simulink model "FOC_control"  (R2019a)
settings: Solver=VariableStepAuto  StartTime=0.0  StopTime=10.0  RelTol=1e-3
undefined symbols (not defined in the file or in its folder): PWM_EN, sf, Ts
libraries: nesl_utility x13, ee_lib x10, fl_lib x10, msbAdcArchitectures x6, eeTransforms x4, eePmsmCurrentController x1, eePmsmCurrentReferenceGen x1, eePwmGeneratorTwoLevel x1, eeVelocityController x1, simulink x1
(part 2 of 3)

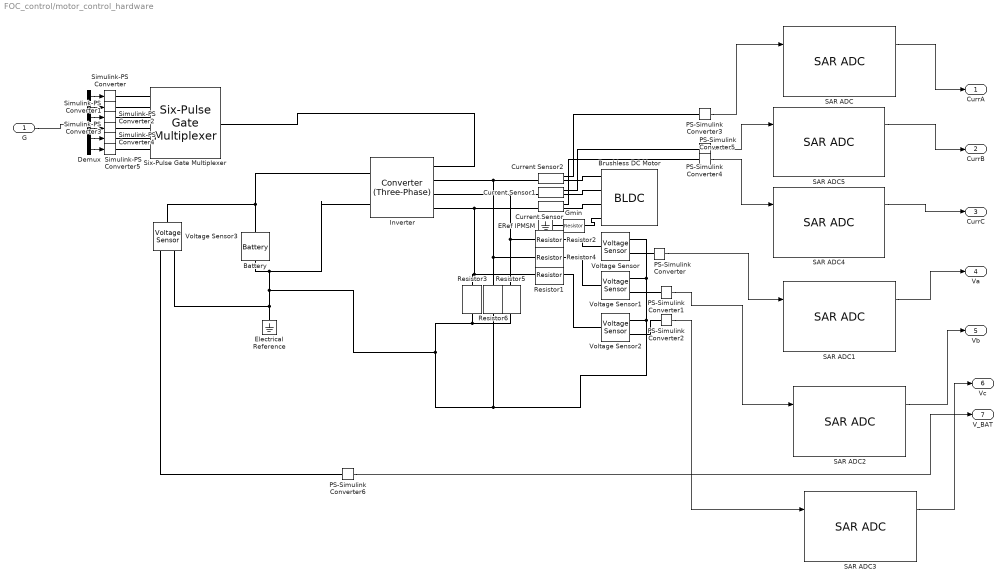
== system FOC_control/motor_control_hardware  ==
  G : Inport  Tag=G
  Battery : ee_lib/Sources/Battery  Vnom=43.2 V  R1=2 Ohm  prm_AH=1  AH=50 hr*A  V1=11.5 V  AH1=25 hr*A  prm_R2=1  R2=2000 Ohm  prm_dyn=1  Rp1=0.005 Ohm  tau1=30 s  Rp2=0.005 Ohm  tau2=30 s  Rp3=0.005 Ohm  tau3=30 s  Rp4=0.005 Ohm  tau4=30 s  Rp5=0.005 Ohm  tau5=30 s  prm_fade=1  N_fade=100  AH_fade=45 hr*A  R1_fade=2.02 Ohm  V1_fade=10.35 V  i_specify=off  i_priority=None  i=0 A  i_nominal_specify=off  i_nominal_unit=A  i_nominal_value=1  v_specify=off  v_priority=None  v=0 V  v_nominal_specify=off  v_nominal_unit=V  v_nominal_value=1  charge_specify=off  charge_priority=High  charge=50 hr*A  charge_nominal_specify=off  charge_nominal_unit=hr*A  charge_nominal_value=1  num_cycles_specify=off  num_cycles_priority=High  num_cycles=0  num_cycles_nominal_specify=off  num_cycles_nominal_unit=1  num_cycles_nominal_value=1  thermal_mass=30000 J/K  Tmeas=298.15 K  Vnom_T2=12 V  R1_T2=2.2 Ohm  V1_T2=11.4 V  R2_T2=2200 Ohm  Rp1_T2=0.005 Ohm  tau1_T2=30 s  Rp2_T2=0.005 Ohm  tau2_T2=30 s  Rp3_T2=0.005 Ohm  tau3_T2=30 s  Rp4_T2=0.005 Ohm  tau4_T2=30 s  Rp5_T2=0.005 Ohm  tau5_T2=30 s  Tmeas2=273.15 K  temperature_specify=off  temperature_priority=High  temperature=298.15 K  temperature_nominal_specify=off  temperature_nominal_unit=K  temperature_nominal_value=1
      settings: SourceProductName=Simscape Electrical
  Brushless DC Motor : ee_lib/Electromechanical/Permanent Magnet/BLDC  rotor_param=1  pm_flux_linkage=0.03 Wb  theta_constant=pi / 12 rad  emf_max=9.6 V  DphiDtheta_tab=[0, -.1528, -.1528, .1528, .1528, 0] Wb/rad  back_emf_tab=[0, -9.6, -9.6, 9.6, 9.6, 0] V  rotor_angle_tab=[0, 7.5, 22.5, 37.5, 52.5, 60] deg  w_meas=600 rpm  nPolePairs=6  stator_param=1  Ld=0.00022 H  Lq=0.00022 H  L0=0.00016 H  Ls=0.0002 H  Lm=0 H  Ms=0.00002 H  Rs=0.013 Ohm  zero_sequence=ee.enum.park.zerosequence.include  J=0.01 kg*m^2  lam=0 N*m/(rad/s)  axes_param=2  i_d_specify=off  i_d_priority=None  i_d=0 A  i_d_nominal_specify=off  i_d_nominal_unit=A  i_d_nominal_value=1  i_q_specify=off  i_q_priority=None  i_q=0 A  i_q_nominal_specify=off  i_q_nominal_unit=A  i_q_nominal_value=1  torque_specify=off  torque_priority=None  torque=0 N*m  torque_nominal_specify=off  torque_nominal_unit=N*m  torque_nominal_value=1  angular_velocity_specify=off  angular_velocity_priority=High  angular_velocity=0 rpm  angular_velocity_nominal_specify=off  angular_velocity_nominal_unit=rpm  angular_velocity_nominal_value=1  angular_position_specify=off  angular_position_priority=High  angular_position=0 deg  angular_position_nominal_specify=off  angular_position_nominal_unit=deg  angular_position_nominal_value=1
      settings: SourceProductName=Simscape Electrical  SourceProductBaseCode=PS
  Current Sensor : fl_lib/Electrical/Electrical Sensors/Current Sensor
  Current Sensor1 : fl_lib/Electrical/Electrical Sensors/Current Sensor
  Current Sensor2 : fl_lib/Electrical/Electrical Sensors/Current Sensor
  Demux : Demux  Outputs=6
  ERef IPMSM : fl_lib/Electrical/Electrical Elements/Electrical Reference
      settings: SourceProductName=Foundation Library
  Electrical Reference : fl_lib/Electrical/Electrical Elements/Electrical Reference
  Gmin : fl_lib/Electrical/Electrical Elements/Resistor  R=1e9 Ohm  i_specify=off  i_priority=High  i=0 A  i_nominal_specify=off  i_nominal_unit=A  i_nominal_value=1  v_specify=off  v_priority=High  v=0 V  v_nominal_specify=off  v_nominal_unit=V  v_nominal_value=1
      settings: SourceProductName=Foundation Library
  Inverter : ee_lib/Semiconductors & Converters/Converters/Converter (Three-Phase)  device_type=4  Vf=0.8 V  Ron=0.001 Ohm  Rds=0.001 Ohm  Goff=1e-5 1/Ohm  Vth=0.5 V  Vgt=1 V  Vgt_off=-1 V  Ih=1 A  diode_param=2  diode_Vf=0.8 V  diode_Ron=0.001 Ohm  diode_Goff=1e-5 1/Ohm  diode_C=50 nF  diode_iRM=-235 A  diode_iF=300 A  diode_idot=-50 A/us  diode_trr_param=1  diode_trr_factor=3  diode_trr=15 us  diode_Qrr=1.5e+3 s*uA  snubber_type=0  Rs=0.1 Ohm  Cs=1e-7 F
      settings: SourceProductName=Simscape Electrical  SourceProductBaseCode=PS
  PS-Simulink Converter{,1..6} (7 alike) : nesl_utility/PS-Simulink Converter  PhysicalDomain=network_engine_domain  SubClassName=ps_output  LeftPortType=input  RightPortType=output  PseudoPeriodic=off  Frequencies=[]  Unit=1  AffineConversion=off
  Resistor1 : ee_lib/Passive/Resistor  R=39000 Ohm  R_tol=1  enable_R_tol=1  tol_distribution=1  nSigma=4  enable_operating_limits=0  operating_limit_action=2  max_working_voltage=100 V  power_rating=1 W  enable_faults=0  fault_action=1  R_faulted=inf Ohm  enable_temporal_fault=0  t_fault=1 s  enable_behavioral_fault=0  max_permissible_current=1 A  t_fail_on_current=1 s  noise_mode=0  sample_time=1e-3 s  repeatability=1  auto_seed=797911566  user_seed=0  Tdevice=25 degC  alpha=3.93e-3 1/K  Tmeas=25 degC  thermal_mass=100 J/K  power_derating_T1=70 degC  power_derating_T2=155 degC  operating_temperature_range_vec=[-50, 150] degC  temperature_specify=off  temperature_priority=High  temperature=298.15 K  temperature_nominal_specify=off  temperature_nominal_unit=K  temperature_nominal_value=1
      settings: SourceProductName=Simscape Electrical
  Resistor2 : ee_lib/Passive/Resistor  R=39000 Ohm  R_tol=1  enable_R_tol=1  tol_distribution=1  nSigma=4  enable_operating_limits=0  operating_limit_action=2  max_working_voltage=100 V  power_rating=1 W  enable_faults=0  fault_action=1  R_faulted=inf Ohm  enable_temporal_fault=0  t_fault=1 s  enable_behavioral_fault=0  max_permissible_current=1 A  t_fail_on_current=1 s  noise_mode=0  sample_time=1e-3 s  repeatability=1  auto_seed=770095556  user_seed=0  Tdevice=25 degC  alpha=3.93e-3 1/K  Tmeas=25 degC  thermal_mass=100 J/K  power_derating_T1=70 degC  power_derating_T2=155 degC  operating_temperature_range_vec=[-50, 150] degC  temperature_specify=off  temperature_priority=High  temperature=298.15 K  temperature_nominal_specify=off  temperature_nominal_unit=K  temperature_nominal_value=1
      settings: SourceProductName=Simscape Electrical
  Resistor3 : ee_lib/Passive/Resistor  R=2200 Ohm  R_tol=1  enable_R_tol=1  tol_distribution=1  nSigma=4  enable_operating_limits=0  operating_limit_action=2  max_working_voltage=100 V  power_rating=1 W  enable_faults=0  fault_action=1  R_faulted=inf Ohm  enable_temporal_fault=0  t_fault=1 s  enable_behavioral_fault=0  max_permissible_current=1 A  t_fail_on_current=1 s  noise_mode=0  sample_time=1e-3 s  repeatability=1  auto_seed=829099697  user_seed=0  Tdevice=25 degC  alpha=3.93e-3 1/K  Tmeas=25 degC  thermal_mass=100 J/K  power_derating_T1=70 degC  power_derating_T2=155 degC  operating_temperature_range_vec=[-50, 150] degC  temperature_specify=off  temperature_priority=High  temperature=298.15 K  temperature_nominal_specify=off  temperature_nominal_unit=K  temperature_nominal_value=1
      settings: SourceProductName=Simscape Electrical
  Resistor4 : ee_lib/Passive/Resistor  R=39000 Ohm  R_tol=1  enable_R_tol=1  tol_distribution=1  nSigma=4  enable_operating_limits=0  operating_limit_action=2  max_working_voltage=100 V  power_rating=1 W  enable_faults=0  fault_action=1  R_faulted=inf Ohm  enable_temporal_fault=0  t_fault=1 s  enable_behavioral_fault=0  max_permissible_current=1 A  t_fail_on_current=1 s  noise_mode=0  sample_time=1e-3 s  repeatability=1  auto_seed=1467350256  user_seed=0  Tdevice=25 degC  alpha=3.93e-3 1/K  Tmeas=25 degC  thermal_mass=100 J/K  power_derating_T1=70 degC  power_derating_T2=155 degC  operating_temperature_range_vec=[-50, 150] degC  temperature_specify=off  temperature_priority=High  temperature=298.15 K  temperature_nominal_specify=off  temperature_nominal_unit=K  temperature_nominal_value=1
      settings: SourceProductName=Simscape Electrical
  Resistor5 : ee_lib/Passive/Resistor  R=2200 Ohm  R_tol=1  enable_R_tol=1  tol_distribution=1  nSigma=4  enable_operating_limits=0  operating_limit_action=2  max_working_voltage=100 V  power_rating=1 W  enable_faults=0  fault_action=1  R_faulted=inf Ohm  enable_temporal_fault=0  t_fault=1 s  enable_behavioral_fault=0  max_permissible_current=1 A  t_fail_on_current=1 s  noise_mode=0  sample_time=1e-3 s  repeatability=1  auto_seed=1289282186  user_seed=0  Tdevice=25 degC  alpha=3.93e-3 1/K  Tmeas=25 degC  thermal_mass=100 J/K  power_derating_T1=70 degC  power_derating_T2=155 degC  operating_temperature_range_vec=[-50, 150] degC  temperature_specify=off  temperature_priority=High  temperature=298.15 K  temperature_nominal_specify=off  temperature_nominal_unit=K  temperature_nominal_value=1
      settings: SourceProductName=Simscape Electrical
  Resistor6 : ee_lib/Passive/Resistor  R=2200 Ohm  R_tol=1  enable_R_tol=1  tol_distribution=1  nSigma=4  enable_operating_limits=0  operating_limit_action=2  max_working_voltage=100 V  power_rating=1 W  enable_faults=0  fault_action=1  R_faulted=inf Ohm  enable_temporal_fault=0  t_fault=1 s  enable_behavioral_fault=0  max_permissible_current=1 A  t_fail_on_current=1 s  noise_mode=0  sample_time=1e-3 s  repeatability=1  auto_seed=4006765953  user_seed=0  Tdevice=25 degC  alpha=3.93e-3 1/K  Tmeas=25 degC  thermal_mass=100 J/K  power_derating_T1=70 degC  power_derating_T2=155 degC  operating_temperature_range_vec=[-50, 150] degC  temperature_specify=off  temperature_priority=High  temperature=298.15 K  temperature_nominal_specify=off  temperature_nominal_unit=K  temperature_nominal_value=1
      settings: SourceProductName=Simscape Electrical
  SAR ADC : msbAdcArchitectures/SAR ADC  DACVoltages=[-5:5]  DACINLVoltages=tanh([-5:5])  NBits=12  InputRange=[-3.3 3.3]  ExtStartClk=on  StartFreq=10e3  StartClkJitter=0  SARFreq=2e7  OutDataType=BinaryVector  EnableImp=on  OffsetError=1  GainError=2  GainErrorUnit=LSB  INL=[1 1.00048851978505 1.0009770395701 1.00146555935515 1.00195407914021 1.00244259892526 1.00293111871031 1.00341963849536 1.00390815828041 1.00439667806546 1.00488519785051 1.00537371763556 1.00586223742062 1.00635075720567 1.00683927699072 1.00732779677577 1.00781631656082 1.00830483634587 1.00879335613092 1.00928187591597 1.00977039570103 1.01025891548608 1.01074743527113 1.01123595505618 1.01172447484123 1.01221299462628 1.01270151441133 1.01319003419638 1.01367855398144 1.01416707376649 1.01465559355154 1.01514411333659 1.01563263312164 1.01612115290669 1.01660967269174 1.01709819247679 1.01758671226185 1.0180752320469 1.01856375183195 1.019052271617 1.01954079140205 1.0200293111871 1.02051783097215 1.0210063507572 1.02149487054226 1.02198339032731 1.02247191011236 1.02296042989741 1.02344894968246 1.02393746946751 1.02442598925256 1.02491450903761 1.02540302882267 1.02589154860772 1.02638006839277 1.02686858817782 1.02735710796287 1.02784562774792 1.02833414753297 1.02882266731802 1.02931118710308 1.02979970688813 1.03028822667318 1.03077674645823 1.03126526624328 1.03175378602833 1.03224230581338 1.03273082559843 1.03321934538349 1.03370786516854 1.03419638495359 1.03468490473864 1.03517342452369 1.03566194430874 1.03615046409379 1.03663898387885 1.0371275036639 1.03761602344895 1.038104543234 1.03859306301905 1.0390815828041 1.03957010258915 1.0400586223742 1.04054714215926 1.04103566194431 1.04152418172936 1.04201270151441 1.04250122129946 1.04298974108451 1.04347826086956 1.04396678065461 1.04445530043967 1.04494382022472 1.04543234000977 1.04592085979482 1.04640937957987 1.04689789936492 1.04738641914997 1.04787493893502 1.04836345872008 1.04885197850513 1.04934049829018 1.04982901807523 1.05031753786028 1.05080605764533 1.05129457743038 1.05178309721543 1.05227161700049 1.05276013678554 1.05324865657059 1.05373717635564 1.05422569614069 1.05471421592574 1.05520273571079 1.05569125549584 1.0561797752809 1.05666829506595 1.057156814851 1.05764533463605 1.0581338544211 1.05862237420615 1.0591108939912 1.05959941377625 1.06008793356131 1.06057645334636 1.06106497313141 1.06155349291646 1.06204201270151 1.06253053248656 1.06301905227161 1.06350757205666 1.06399609184172 1.06448461162677 1.06497313141182 1.06546165119687 1.06595017098192 1.06643869076697 1.06692721055202 1.06741573033707 1.06790425012213 1.06839276990718 1.06888128969223 1.06936980947728 1.06985832926233 1.07034684904738 1.07083536883243 1.07132388861748 1.07181240840254 1.07230092818759 1.07278944797264 1.07327796775769 1.07376648754274 1.07425500732779 1.07474352711284 1.0752320468979 1.07572056668295 1.076209086468 1.07669760625305 1.0771861260381 1.07767464582315 1.0781631656082 1.07865168539325 1.07914020517831 1.07962872496336 1.08011724474841 1.08060576453346 1.08109428431851 1.08158280410356 1.08207132388861 1.08255984367366 1.08304836345872 1.08353688324377 1.08402540302882 1.08451392281387 1.08500244259892 1.08549096238397 1.08597948216902 1.08646800195407 1.08695652173913 1.08744504152418 1.08793356130923 1.08842208109428 1.08891060087933 1.08939912066438 1.08988764044943 1.09037616023448 1.09086468001954 1.09135319980459 1.09184171958964 1.09233023937469 1.09281875915974 1.09330727894479 1.09379579872984 1.09428431851489 1.09477283829995 1.095261358085 1.09574987787005 1.0962383976551 1.09672691744015 1.0972154372252 1.09770395701025 1.0981924767953 1.09868099658036 1.09916951636541 1.09965803615046 1.10014655593551 1.10063507572056 1.10112359550561 1.10161211529066 1.10210063507571 1.10258915486077 1.10307767464582 1.10356619443087 1.10405471421592 1.10454323400097 1.10503175378602 1.10552027357107 1.10600879335612 1.10649731314118 1.10698583292623 1.10747435271128 1.10796287249633 1.10845139228138 1.10893991206643 1.10942843185148 1.10991695163654 1.11040547142159 1.11089399120664 1.11138251099169 1.11187103077674 1.11235955056179 1.11284807034684 1.11333659013189 1.11382510991695 1.114313629702 1.11480214948705 1.1152906692721 ...(+65139 chars)]
      settings: SourceProductName=Mixed-Signal Blockset  SourceProductBaseCode=AM
  SAR ADC{1..5} (5 alike) : msbAdcArchitectures/SAR ADC  DACVoltages=[-5:5]  DACINLVoltages=tanh([-5:5])  NBits=8  InputRange=[-1 1]  ExtStartClk=on  StartFreq=10e3  StartClkJitter=0  SARFreq=2e7  OutDataType=BinaryVector  EnableImp=on  OffsetError=1  GainError=2  GainErrorUnit=LSB  INL=[1 1.00787401574803 1.01574803149606 1.02362204724409 1.03149606299213 1.03937007874016 1.04724409448819 1.05511811023622 1.06299212598425 1.07086614173228 1.07874015748031 1.08661417322835 1.09448818897638 1.10236220472441 1.11023622047244 1.11811023622047 1.1259842519685 1.13385826771654 1.14173228346457 1.1496062992126 1.15748031496063 1.16535433070866 1.17322834645669 1.18110236220473 1.18897637795276 1.19685039370079 1.20472440944882 1.21259842519685 1.22047244094488 1.22834645669291 1.23622047244094 1.24409448818898 1.25196850393701 1.25984251968504 1.26771653543307 1.2755905511811 1.28346456692913 1.29133858267716 1.2992125984252 1.30708661417323 1.31496062992126 1.32283464566929 1.33070866141733 1.33858267716536 1.34645669291339 1.35433070866141 1.36220472440945 1.37007874015748 1.37795275590551 1.38582677165354 1.39370078740158 1.40157480314961 1.40944881889764 1.41732283464567 1.4251968503937 1.43307086614173 1.44094488188976 1.44881889763779 1.45669291338583 1.46456692913386 1.47244094488189 1.48031496062992 1.48818897637796 1.49606299212599 1.50393700787401 1.51181102362204 1.51968503937007 1.5275590551181 1.53543307086615 1.54330708661418 1.55118110236221 1.55905511811024 1.56692913385827 1.5748031496063 1.58267716535433 1.59055118110236 1.5984251968504 1.60629921259843 1.61417322834646 1.62204724409449 1.62992125984252 1.63779527559055 1.64566929133858 1.65354330708661 1.66141732283465 1.66929133858268 1.67716535433071 1.68503937007874 1.69291338582677 1.7007874015748 1.70866141732283 1.71653543307086 1.7244094488189 1.73228346456693 1.74015748031496 1.74803149606299 1.75590551181102 1.76377952755905 1.77165354330708 1.77952755905511 1.78740157480316 1.79527559055119 1.80314960629921 1.81102362204724 1.81889763779527 1.8267716535433 1.83464566929133 1.84251968503936 1.85039370078741 1.85826771653544 1.86614173228347 1.8740157480315 1.88188976377953 1.88976377952756 1.89763779527559 1.90551181102362 1.91338582677166 1.92125984251969 1.92913385826772 1.93700787401575 1.94488188976378 1.95275590551181 1.96062992125984 1.96850393700787 1.97637795275591 1.98425196850394 1.99212598425197 2 2.00787401574803 2.01574803149606 2.02362204724409 2.03149606299212 2.03937007874015 2.04724409448818 2.05511811023621 2.06299212598427 2.0708661417323 2.07874015748033 2.08661417322836 2.09448818897638 2.10236220472441 2.11023622047244 2.11811023622047 2.1259842519685 2.13385826771653 2.14173228346456 2.14960629921259 2.15748031496062 2.16535433070865 2.17322834645668 2.18110236220471 2.18897637795277 2.1968503937008 2.20472440944883 2.21259842519686 2.22047244094489 2.22834645669292 2.23622047244095 2.24409448818898 2.25196850393701 2.25984251968504 2.26771653543307 2.2755905511811 2.28346456692913 2.29133858267716 2.29921259842519 2.30708661417322 2.31496062992127 2.3228346456693 2.33070866141733 2.33858267716536 2.34645669291339 2.35433070866142 2.36220472440945 2.37007874015748 2.37795275590551 2.38582677165354 2.39370078740157 2.4015748031496 2.40944881889763 2.41732283464566 2.42519685039369 2.43307086614172 2.44094488188978 2.44881889763781 2.45669291338584 2.46456692913387 2.4724409448819 2.48031496062993 2.48818897637796 2.49606299212599 2.50393700787401 2.51181102362204 2.51968503937007 2.5275590551181 2.53543307086613 2.54330708661416 2.55118110236219 2.55905511811022 2.56692913385828 2.57480314960631 2.58267716535434 2.59055118110237 2.5984251968504 2.60629921259843 2.61417322834646 2.62204724409449 2.62992125984252 2.63779527559055 2.64566929133858 2.65354330708661 2.66141732283464 2.66929133858267 2.6771653543307 2.68503937007873 2.69291338582678 2.70078740157481 2.70866141732284 2.71653543307087 2.7244094488189 2.73228346456693 2.74015748031496 2.74803149606299 2.75590551181102 2.76377952755905 2.77165354330708 2.77952755905511 2.78740157480314 2.79527559055117 2.8031496062992 2.81102362204723 2.81889763779529 2.82677165354332 2.83464566929135 2.84251968503938 2.85039370078741 2.85826771653544 2.86614173228347 2.8740157480315 2.88188976377953 2.88976377952756 2.89763779527559 2.90551181102362 2.91338582677164 2.92125984251967 2.9291338582677 2.93700787401573 2.94488188976379 2.95275590551182 2.96062992125985 2.96850393700788 2.97637795275591 2.98425196850394 2.99212598425197 3]
      settings: SourceProductName=Mixed-Signal Blockset  SourceProductBaseCode=AM
  Simulink-PS Converter{,1..5} (6 alike) : nesl_utility/Simulink-PS Converter  PhysicalDomain=network_engine_domain  SubClassName=ps_input  LeftPortType=input  RightPortType=output  PseudoPeriodic=off  Frequencies=[]  NoiseDistribution=none  NoiseParameters=[]  Unit=1  AffineConversion=off  FilteringAndDerivatives=provide  SimscapeFilterOrder=1  InputFilterTimeConstant=0.001  UdotUserProvided=0
  Six-Pulse Gate Multiplexer : ee_lib/Semiconductors & Converters/Converters/Six-Pulse Gate Multiplexer  R=0 Ohm
      settings: SourceProductName=Simscape Electrical  SourceProductBaseCode=PS
  Voltage Sensor{,1..3} (4 alike) : fl_lib/Electrical/Electrical Sensors/Voltage Sensor
  "CurrA " : Outport
  "CurrB " : Outport  Port=2
  "CurrC " : Outport  Port=3
  "Va " : Outport  Port=4
  "Vb " : Outport  Port=5
  "Vc " : Outport  Port=6
  "V_BAT " : Outport  Port=7
  wires:
  G/1 -> Demux/1
  Demux/1 -> Simulink-PS Converter/1
  Demux/2 -> Simulink-PS Converter1/1
  Demux/3 -> Simulink-PS Converter2/1
  Demux/4 -> Simulink-PS Converter3/1
  Demux/5 -> Simulink-PS Converter4/1
  Demux/6 -> Simulink-PS Converter5/1
  PS-Simulink Converter/1 -> SAR ADC1/1
  PS-Simulink Converter1/1 -> SAR ADC2/1
  PS-Simulink Converter2/1 -> SAR ADC3/1
  PS-Simulink Converter3/1 -> SAR ADC/1
  PS-Simulink Converter4/1 -> SAR ADC5/1
  PS-Simulink Converter5/1 -> SAR ADC4/1
  SAR ADC5/1 -> "CurrB "/1
  SAR ADC2/1 -> "Vb "/1
  SAR ADC3/1 -> "Vc "/1
  SAR ADC/1 -> "CurrA "/1
  SAR ADC1/1 -> "Va "/1
  SAR ADC4/1 -> "CurrC "/1
  PS-Simulink Converter6/1 -> "V_BAT "/1
  connections:
  Inverter/LConn3 -- Current Sensor1/LConn1 -- Resistor5/LConn1 -- Resistor2/LConn1
  Inverter/LConn4 -- Resistor3/LConn1 -- Resistor1/LConn1 -- Current Sensor/LConn1
  Inverter/LConn2 -- Current Sensor2/LConn1 -- Resistor6/LConn1 -- Resistor4/LConn1
  Simulink-PS Converter3/RConn1 -- Six-Pulse Gate Multiplexer/LConn4
  Simulink-PS Converter4/RConn1 -- Six-Pulse Gate Multiplexer/LConn5
  Simulink-PS Converter5/RConn1 -- Six-Pulse Gate Multiplexer/LConn6
  Simulink-PS Converter2/RConn1 -- Six-Pulse Gate Multiplexer/LConn3
  Simulink-PS Converter1/RConn1 -- Six-Pulse Gate Multiplexer/LConn2
  Simulink-PS Converter/RConn1 -- Six-Pulse Gate Multiplexer/LConn1
  Six-Pulse Gate Multiplexer/RConn1 -- Inverter/LConn1
  Battery/LConn1 -- Voltage Sensor3/LConn1 -- Inverter/RConn1
  Battery/RConn1 -- Voltage Sensor3/RConn2 -- Electrical Reference/LConn1 -- Voltage Sensor1/RConn2 -- Voltage Sensor/RConn2 -- Voltage Sensor2/RConn2 -- Resistor6/RConn1 -- Resistor5/RConn1 -- Resistor3/RConn1 -- Inverter/RConn2
  Voltage Sensor/LConn1 -- Resistor2/RConn1
  Voltage Sensor/RConn1 -- PS-Simulink Converter/LConn1
  Resistor4/RConn1 -- Voltage Sensor1/LConn1
  Resistor1/RConn1 -- Voltage Sensor2/LConn1
  Voltage Sensor1/RConn1 -- PS-Simulink Converter1/LConn1
  PS-Simulink Converter2/LConn1 -- Voltage Sensor2/RConn1
  Gmin/RConn1 -- Brushless DC Motor/LConn4
  ERef IPMSM/LConn1 -- Gmin/LConn1
  Current Sensor/RConn2 -- Brushless DC Motor/LConn3
  Current Sensor1/RConn2 -- Brushless DC Motor/LConn2
  Current Sensor2/RConn2 -- Brushless DC Motor/LConn1
  PS-Simulink Converter3/LConn1 -- Current Sensor2/RConn1
  PS-Simulink Converter4/LConn1 -- Current Sensor1/RConn1
  PS-Simulink Converter5/LConn1 -- Current Sensor/RConn1
  Voltage Sensor3/RConn1 -- PS-Simulink Converter6/LConn1
